simulink model "hinf_swarm_single"  (R2025a)
settings: Solver=VariableStepAuto  StartTime=0.0  StopTime=60  RelTol=1e-6
PostLoadFcn:
  | init.m
values from neighbouring files (symbols this model uses):
  A = [0 0 0 0 0 0 -g 0 0 0 0 0 ... (first row only)    [analysis.m]    (also in constants.m; hinf_design.m; linear_nonlinear_comparison.m)
  B = [0 0 0 0 ... (first row only)    [analysis.m]    (also in constants.m; hinf_design.m; linear_nonlinear_comparison.m)
  simcase = STABILIZE    (= 4)    [analysis.m]    (also in sweep_ballistic_envelope.m; sweep_landing_centroid.m)
  x0_step = [2; 4; 10]    [analysis.m]    (also in sweep_ballistic_envelope.m; sweep_landing_centroid.m)
  xf = [2; 4; 10]    [analysis.m]    (also in sweep_ballistic_envelope.m = [0; 0; 0]; sweep_landing_centroid.m = [0; 0; 0])
  xf_ballistic = [xi(10:11,:);0]    [analysis.m]    (also in sweep_ballistic_envelope.m = [xi(10:11); 0]; sweep_landing_centroid.m = land_pos(:, target_idx, k))
  xi = [vel0; rotvel0; rot0; x0]    [analysis.m]    (also in ballistic_deploy_state.m = [vel0; rotvel0; theta0; phi0; psi0; pos_nwu]; dsmc_constraints.m = (1 - k_xi) .* xi + delta_u; forensic_envelope.m = ballistic_deploy_state(dp(1:3), dp(4:6), dp(7:9), dp(10:12)); sweep_ballistic_envelope.m = ballistic_deploy_state(deploy_point(1:3), deploy_point(4:6),)
libraries: uavutilslib x1
settings Model: SimulationMode=rapid-accelerator  ExtModeTrigDuration=100  Creator=johnpye  LastModifiedBy=johnpye

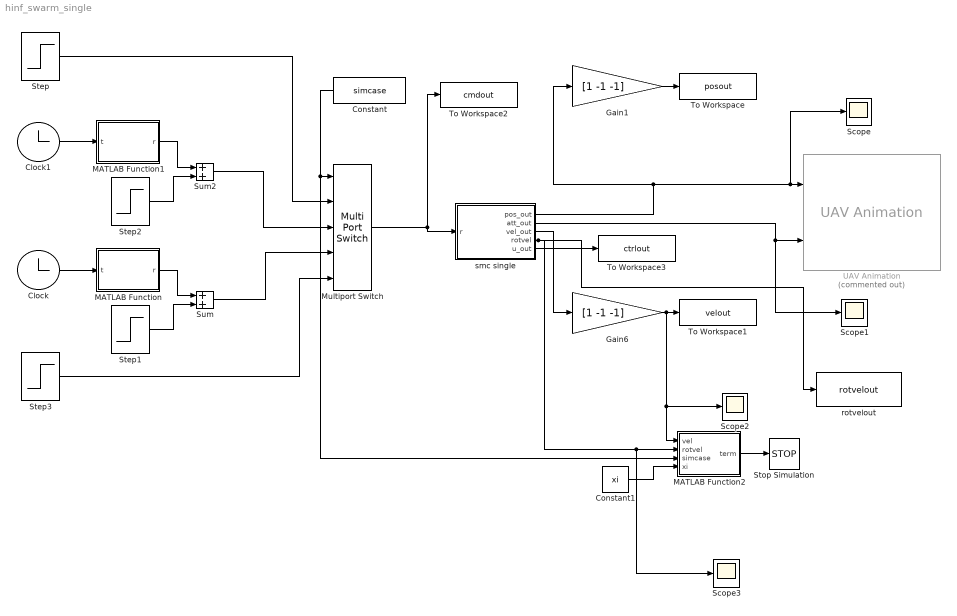
== system hinf_swarm_single ==
  Clock : Clock
  Clock1 : Clock
  Constant : Constant  Value=simcase
  Constant1 : Constant  Value=xi
  Gain1 : Gain  Gain=[1 -1 -1]
  Gain6 : Gain  Gain=[1 -1 -1]
  MATLAB Function : MATLAB Function  TreatAsAtomicUnit=on
  MATLAB Function1 : MATLAB Function  TreatAsAtomicUnit=on
  MATLAB Function2 : MATLAB Function  TreatAsAtomicUnit=on
  Multiport Switch : MultiPortSwitch  Inputs=4  SaturateOnIntegerOverflow=off  InputSameDT=off
  Scope{,1..3} (4 alike) : Scope
      Scope settings: ActiveDisplayYMinimum=-140.6410815383484  ActiveDisplayYMaximum=1005.2301529089905  DataLoggingVariableName=ScopeData9
      Scope1 settings: ActiveDisplayYMinimum=-0.39814584953510085  ActiveDisplayYMaximum=0.3797080874392163
      Scope2 settings: ActiveDisplayYMinimum=-18.885536263073504  ActiveDisplayYMaximum=111.94870875985907
      Scope3 settings: ActiveDisplayYMinimum=-139418.85945896356  ActiveDisplayYMaximum=35259.804825236613  DataLoggingVariableName=ScopeData2
  Step : Step  Time=0  Before=x0_step  After=xf  SampleTime=0  VectorParams1D=off
  Step1 : Step  Time=0  Before=[0; 0; 0]  After=[0; 0; 10]  SampleTime=0  VectorParams1D=off
  Step2 : Step  Time=0  Before=[0; 0; 0]  After=[0; 0; 10]  SampleTime=0  VectorParams1D=off
  Step3 : Step  Time=0  Before=xi(10:12,:)  After=xf_ballistic  SampleTime=0  VectorParams1D=off
  Stop Simulation : Stop
  Sum : Sum
  Sum2 : Sum
  To Workspace : ToWorkspace  VariableName=posout  SaveFormat=Timeseries  SampleTime=-1
  To Workspace1 : ToWorkspace  VariableName=velout  SaveFormat=Timeseries  SampleTime=-1
  To Workspace2 : ToWorkspace  VariableName=cmdout  SaveFormat=Timeseries  SampleTime=-1
  To Workspace3 : ToWorkspace  VariableName=ctrlout  SaveFormat=Timeseries  SampleTime=-1
  UAV Animation : uavutilslib/UAV Animation  Commented=on  NumUAV=1  DynamicUAVConfig=off  UAVType=Multirotor  UAVSize=1  UAVColor=[1 0 0]  UAVTrajectoryAlpha=1  InertialZDirection=Down  RotationFormat=Euler ZYX  DrawMarkers=off  SampleTime=0.01
  rotvelout : ToWorkspace  VariableName=rotvelout  SaveFormat=Timeseries  SampleTime=-1
  smc single : Subsystem
  wires:
  smc single/2(att_out) -> Scope1/1, UAV Animation/2
  smc single/1(pos_out) -> Gain1/1, Scope/1, UAV Animation/1
  Multiport Switch/1 -> To Workspace2/1, smc single/1(r)
  Gain1/1 -> To Workspace/1
  Gain6/1 -> MATLAB Function2/1(vel), Scope2/1, To Workspace1/1
  smc single/3(vel_out) -> Gain6/1
  Constant/1 -> MATLAB Function2/3(simcase), Multiport Switch/1
  Sum/1 -> Multiport Switch/4
  Step3/1 -> Multiport Switch/5
  Step2/1 -> Sum2/2
  MATLAB Function/1(r) -> Sum/1
  Step/1 -> Multiport Switch/2
  Clock1/1 -> MATLAB Function1/1(t)
  Clock/1 -> MATLAB Function/1(t)
  MATLAB Function1/1(r) -> Sum2/1
  Sum2/1 -> Multiport Switch/3
  Step1/1 -> Sum/2
  MATLAB Function2/1(term) -> Stop Simulation/1
  smc single/4(rotvel) -> Scope3/1, MATLAB Function2/2(rotvel), rotvelout/1
  Constant1/1 -> MATLAB Function2/4(xi)
  smc single/5(u_out) -> To Workspace3/1

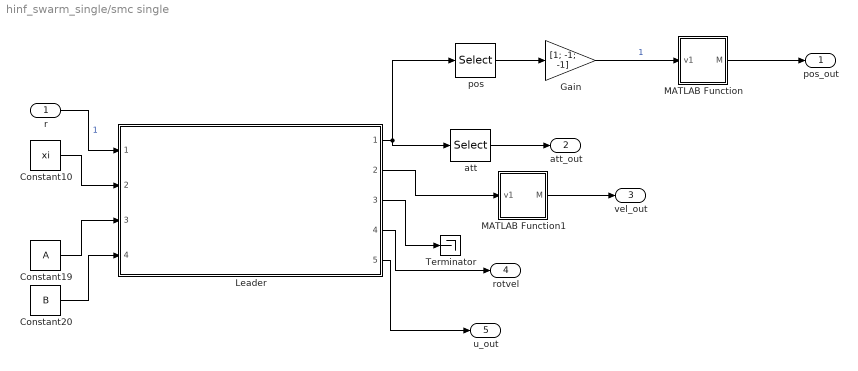
== system hinf_swarm_single/smc single ==
  r : Inport
  Constant10 : Constant  Value=xi
  Constant19 : Constant  Value=A
  Constant20 : Constant  Value=B
  Gain : Gain  Gain=[1; -1; -1]
  Leader : Subsystem  ReferencedSubsystem=actual_hinf_controller
  MATLAB Function : MATLAB Function  TreatAsAtomicUnit=on
  MATLAB Function1 : MATLAB Function  TreatAsAtomicUnit=on
  Terminator : Terminator
  att : Selector  InputPortWidth=12  IndexOptions=Index vector (dialog)  Indices=[7 8 9]  OutputSizes=1
  pos : Selector  InputPortWidth=12  IndexOptions=Index vector (dialog)  Indices=[10 11 12]  OutputSizes=1
  pos_out : Outport
  att_out : Outport  Port=2
  vel_out : Outport  Port=3
  rotvel : Outport  Port=4
  u_out : Outport  Port=5
  wires:
  Leader/1 -> att/1, pos/1
  Gain/1 -> MATLAB Function/1(v1)  "1"
  Leader/2 -> MATLAB Function1/1(v1)
  r/1 -> Leader/1  "1"
  pos/1 -> Gain/1
  Constant10/1 -> Leader/2
  att/1 -> att_out/1
  Leader/3 -> Terminator/1
  Constant20/1 -> Leader/4
  Constant19/1 -> Leader/3
  MATLAB Function/1(M) -> pos_out/1
  MATLAB Function1/1(M) -> vel_out/1
  Leader/4 -> rotvel/1
  Leader/5 -> u_out/1

== matlab function hinf_swarm_single/smc single/MATLAB Function1 ==
  data: v1 input; M output
function M = fcn(v1)

v1 = reshape(v1, [1, 3]);

M = v1;

== matlab function hinf_swarm_single/MATLAB Function2 ==
  data: vel input; term output; rotvel input; simcase input; xi input
function term = fcn(vel,rotvel,simcase,xi)

if simcase == 4
    if norm(vel) >= 10e4 ...
        || norm(rotvel) >= 10e4
        term = 1;
    else
        term = 0;
    end
else
    term = 0;
end

== matlab function hinf_swarm_single/MATLAB Function ==
  data: t input; r output
function r = fcn(t)

r = [0.05*t*cos(2*pi*0.05*t); 0.05*t*sin(2*pi*0.05*t); 0];

== matlab function hinf_swarm_single/MATLAB Function1 ==
  data: t input; r output
function r = fcn(t)

r = [-0.25*cos(2*pi*0.05*t); 10*sin(2*pi*0.05*t)*cos(2*pi*0.05*t); 0];

== matlab function hinf_swarm_single/smc single/MATLAB Function ==
  data: v1 input; M output
function M = fcn(v1)

v1 = reshape(v1, [1, 3]);

M = v1;
